simulink model "feedback_z"  (R2018b)
settings: Solver=VariableStepAuto  StartTime=0.0  StopTime=10  RelTol=1e-3
undefined symbols (not defined in the file): Az, Az_prime, Bz, Bz_prime, Cz, Cz_prime, Dz, Dz_prime, Kz, Sz, x0_chap, x0z
settings Model: Creator=olavoie  LastModifiedBy=Rafik

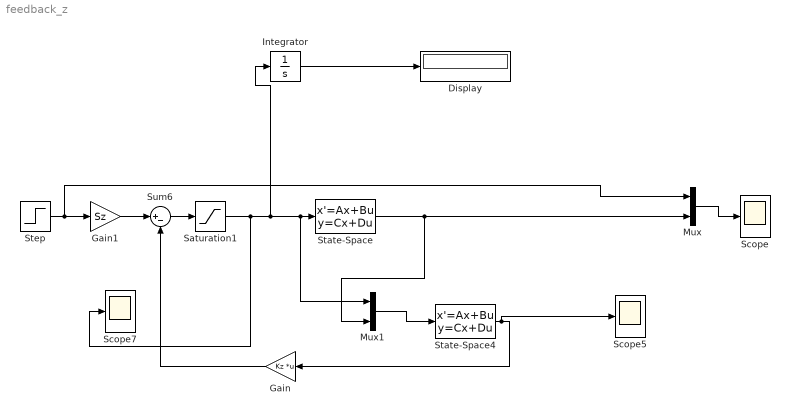
== system feedback_z ==
  Display : Display
  Gain : Gain  Gain=Kz  Multiplication=Matrix(K*u)
  Gain1 : Gain  Gain=Sz
  Integrator : Integrator
  Mux : Mux  Inputs=2
  Mux1 : Mux  Inputs=2
  Saturation1 : Saturate  UpperLimit=110  LowerLimit=-110
  Scope : Scope
  Scope5 : Scope
  Scope7 : Scope
  State-Space : StateSpace  A=Az  B=Bz  C=Cz  D=Dz  InitialCondition=x0z
  State-Space4 : StateSpace  A=Az_prime  B=Bz_prime  C=Cz_prime  D=Dz_prime  InitialCondition=x0_chap
  Step : Step  Time=0  After=0.4  SampleTime=0
  Sum6 : Sum  Inputs=|+-
  wires:
  Sum6/1 -> Saturation1/1
  Mux1/1 -> State-Space4/1
  State-Space/1 -> Mux/2, Mux1/2
  Mux/1 -> Scope/1
  Gain/1 -> Sum6/2
  State-Space4/1 -> Scope5/1, Gain/1
  Step/1 -> Mux/1, Gain1/1
  Gain1/1 -> Sum6/1
  Saturation1/1 -> Scope7/1, Mux1/1, State-Space/1, Integrator/1
  Integrator/1 -> Display/1
